simulink library "dlbsBlockDenseLayer"  (R2025b)
settings: Solver=VariableStepAuto  StartTime=0.0  StopTime=10.0  RelTol=1e-3
libraries: dlbsBlockAdd x1, dlbsBlockMatrixMultiply x1
settings Model: Creator=lt6037  LastModifiedBy=lt6037

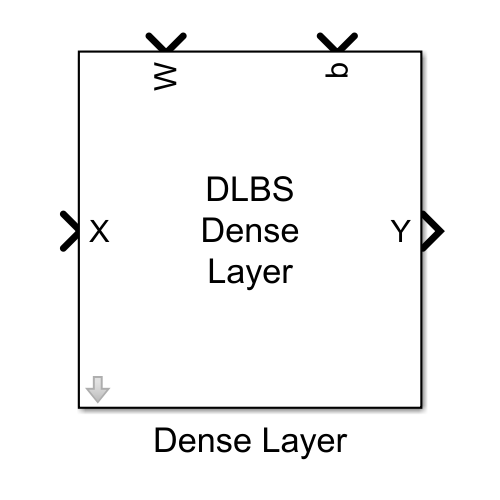
[thumbnail: Simulink's stored preview of the top-level diagram]
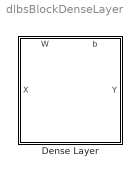
== system dlbsBlockDenseLayer ==
  Dense Layer : Subsystem
      mask help: The Dense Layer block implements a fully connected layer, which is a fundamental building block in many neural network architectures. It performs a linear transformation of the input data followed by an optional activation function.
      settings: PortSchema="{\"entries\":[{\"content\":{\"sides\":[{\"content\":{\"connectorIds\":[\"In1\"]},\"type\":\"ConnectorPlacement.EquallySpacedRectSide\",\"uuid\":\"b33e3efa-c5b8-41d4-b1ca-cb1849ea98a3\"},{\"content\":{\"connectorIds\":[\"Out1\"],\"side\":\"RIGHT\"},\"type\":\"ConnectorPlacement.EquallySpacedRectSide\",\"uuid\":\"a0e24e36-46d7-46cd-ac82-63f9632b3759\"},{\"content\":{\"connectorIds\":[\"In2\",\"In3\"],\"side\":\"TOP\"},\"type\":\"ConnectorPlacement.EquallySpacedRectSide\",\"uuid\":\"958bfc09-87b0-4260-b7c0-76314fc0987c\"}]},\"type\":\"ConnectorPlacement.EquallySpacedConnector\",\"uuid\":\"b1e0a12c-b48f-44f5-9961-593225bd0b2c\"}],\"packageUris\":[\"http://schema.mathworks.com/mf0/Connector/R2020b\"],\"version\":\"1.0\"}"
      mask Help: web("dlbsHelpBlockDenseLayer.html")
      mask Display: fprintf("DLBS\nDense\nLayer")

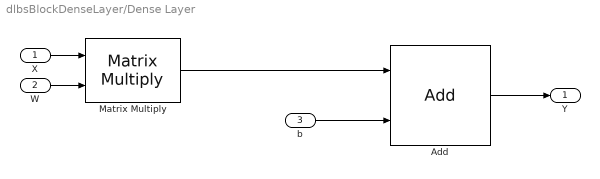
== system dlbsBlockDenseLayer/Dense Layer ==
  X : Inport
  W : Inport  Port=2
  b : Inport  Port=3
  Add : dlbsBlockAdd/Add  LabelModeActiveChoice=broadcast  broadcast=on  dims1=[]  dims2=[1]
  Matrix Multiply : dlbsBlockMatrixMultiply/Matrix Multiply
  Y : Outport
  wires:
  Matrix Multiply/1 -> Add/1
  X/1 -> Matrix Multiply/1
  W/1 -> Matrix Multiply/2
  b/1 -> Add/2
  Add/1 -> Y/1
